simulink model "VCMGCM1962020b_v2"  (R2020b)
settings: Solver=FixedStepDiscrete  StartTime=0.0  StopTime=10.0  FixedStep=0.005  RelTol=1e-3  EnableMultiTasking=on
PreLoadFcn:
  | try, model_open; catch, disp('Error occurred while executing model pre-load callback: model_open.m'); disp('Please assure that the MATLAB working directory is set to the model directory before opening.'); end
InitFcn:
  | try, model_open; catch, end
undefined symbols (not defined in the file): Bridge, GCM, H, raptor_get_param_eval, raptor_get_safe_string, raptor_xcp_function
libraries: Blocks_lib x1165, Raptor_lib x665, simulink x62, VCM_lib x5
(part 19 of 23)

== system VCMGCM1962020b_v2/Fgnd/Sensors/CAN/Other/EPAS/EPASG7GenericFdbk2 ==
  DiagEnbl : Inport
  Bus Creator : BusCreator  Inputs=4
  CANRxField : Blocks_lib/CANRxField  typ='double'  custom=off  custom_nam=[nam '---']  custom_units='---'
  CANRxField1 : Blocks_lib/CANRxField  typ='double'  custom=off  custom_nam=[nam '---']  custom_units='---'
  CANRxField2 : Blocks_lib/CANRxField  typ='double'  custom=off  custom_nam=[nam '---']  custom_units='---'
  CANRxMsgStatus : Blocks_lib/CANRxMsgStatus  samptime=samptime  custom=on  custom_nam=[nam '---']  msgnam=EPASG7GenericFdbk2
  Header : Blocks_lib/Header  width=Landscape  addtext=''
  raptor_can_rxmsg : Raptor_lib/CAN/raptor_can_rxmsg  canDefinition=struct('dbcFile', 'EPAS_G7GenericExternal.dbc','message', 'G7GenericFdbk2','comment', '','signals', {{'FDBK2_Velocity','FDBK2_MotorTemperature','FDBK2_BoardTemperature'}},'enabled', [ 1 1 1;],'scaled', [ 1 1 1;],'canBus', 'bus','messageID', [ 419365651;],'idMask', [ 536870911;],'payloadMask', [],'payloadValue', [],'period', [ 0;],'mailbox', '[]','queueSize', [ 1;],'label', [ 1;],'ver', [ 2;],'showID', [ 0;],'showRaw', [ 0;],'fill', [ 0;],'editID', [ 0;],'signalOrder', [ 3;],'signalAscDes', [ 1;])  canBus=bus  mailbox=[]  payloadMask=[]  payloadValue=[]  idMask=hex2dec('1FFFFFFF')  queueSize=1  showID=0  label=1  fill=0  id=419365651  showRaw=0  showAge=1  signalOrder=3  signalInfo={{struct('Name', 'FDBK2_Velocity','Startbit', [ 0;],'SignalSize', [ 32;],'ByteOrder', 'LittleEndian','ValueType', 'SIGNED','Class', 'int32','Signed', [ 1;],'Factor', [ 9.5367e-07;],'Offset', [ 0;],'Min', [ -2048;],'Max', [ 2048;],'Units', 'RPM','Comment', '','StartBit', [ 0;]),struct('Name', 'FDBK2_MotorTemperature','Startbit', [ 0;],'SignalSize', [ 8;],'ByteOrder', 'LittleEndian','ValueType', 'UNSIGNED','Class', 'uint8','Signed', [ 0;],'Factor', [ 1;],'Offset', [ -40;],'Min', [ -40;],'Max', [ 215;],'Units', 'C','Comment', '','StartBit', [ 48;]),struct('Name', 'FDBK2_BoardTemperature','Startbit', [ 0;],'SignalSize', [ 8;],'ByteOrder', 'LittleEndian','ValueType', 'UNSIGNED','Class', 'uint8','Signed', [ 0;],'Factor', [ 1;],'Offset', [ -40;],'Min', [ -40;],'Max', [ 215;],'Units', 'C','Comment', '','StartBit', [ 32;])}}
      settings: SourceProductName=Raptor
  Data : Outport  VectorParamsAs1DForOutWhenUnconnected=off
  wires:
  Bus Creator/1 -> Data/1  "EPASG7GenericFdbk2"
  raptor_can_rxmsg/2 -> CANRxField/1  "FDBK2_Velocity"
  CANRxMsgStatus/1 -> Bus Creator/1
  CANRxField/1 -> Bus Creator/2
  DiagEnbl/1 -> CANRxMsgStatus/1
  raptor_can_rxmsg/1 -> CANRxMsgStatus/2  "Age"
  raptor_can_rxmsg/3 -> CANRxField1/1  "FDBK2_MotorTemperature"
  CANRxField1/1 -> Bus Creator/3
  raptor_can_rxmsg/4 -> CANRxField2/1  "FDBK2_BoardTemperature"
  CANRxField2/1 -> Bus Creator/4

== system VCMGCM1962020b_v2/Fgnd/Sensors/CAN/Other/EPAS/EPASG7GenericFdbk3 ==
  DiagEnbl : Inport
  Bus Creator : BusCreator  Inputs=3
  CANRxField : Blocks_lib/CANRxField  typ='double'  custom=off  custom_nam=[nam '---']  custom_units='---'
  CANRxField1 : Blocks_lib/CANRxField  typ='double'  custom=off  custom_nam=[nam '---']  custom_units='---'
  CANRxMsgStatus : Blocks_lib/CANRxMsgStatus  samptime=samptime  custom=on  custom_nam=[nam '---']  msgnam=EPASG7GenericFdbk3
  Header : Blocks_lib/Header  width=Landscape  addtext=''
  raptor_can_rxmsg : Raptor_lib/CAN/raptor_can_rxmsg  canDefinition=struct('dbcFile', 'EPAS_G7GenericExternal.dbc','message', 'G7GenericFdbk3','comment', '','signals', {{'FDBK3_TorqueIn','FDBK3_AssistCommand'}},'enabled', [ 1 1;],'scaled', [ 1 1;],'canBus', 'bus','messageID', [ 419365907;],'idMask', [ 536870911;],'payloadMask', [],'payloadValue', [],'period', [ 0;],'mailbox', '[]','queueSize', [ 1;],'label', [ 1;],'ver', [ 2;],'showID', [ 0;],'showRaw', [ 0;],'fill', [ 0;],'editID', [ 0;],'signalOrder', [ 3;],'signalAscDes', [ 1;])  canBus=bus  mailbox=[]  payloadMask=[]  payloadValue=[]  idMask=hex2dec('1FFFFFFF')  queueSize=1  showID=0  label=1  fill=0  id=419365907  showRaw=0  showAge=1  signalOrder=3  signalInfo={{struct('Name', 'FDBK3_TorqueIn','Startbit', [ 0;],'SignalSize', [ 32;],'ByteOrder', 'LittleEndian','ValueType', 'SIGNED','Class', 'int32','Signed', [ 1;],'Factor', [ 9.5367e-07;],'Offset', [ 0;],'Min', [ -2048;],'Max', [ 2048;],'Units', 'Nm','Comment', '','StartBit', [ 0;]),struct('Name', 'FDBK3_AssistCommand','Startbit', [ 0;],'SignalSize', [ 32;],'ByteOrder', 'LittleEndian','ValueType', 'SIGNED','Class', 'int32','Signed', [ 1;],'Factor', [ 9.5367e-07;],'Offset', [ 0;],'Min', [ -2048;],'Max', [ 2048;],'Units', '%','Comment', '','StartBit', [ 32;])}}
      settings: SourceProductName=Raptor
  Data : Outport  VectorParamsAs1DForOutWhenUnconnected=off
  wires:
  CANRxField1/1 -> Bus Creator/3
  raptor_can_rxmsg/3 -> CANRxField1/1  "FDBK3_AssistCommand"
  raptor_can_rxmsg/1 -> CANRxMsgStatus/2  "Age"
  DiagEnbl/1 -> CANRxMsgStatus/1
  CANRxField/1 -> Bus Creator/2
  CANRxMsgStatus/1 -> Bus Creator/1
  raptor_can_rxmsg/2 -> CANRxField/1  "FDBK3_TorqueIn"
  Bus Creator/1 -> Data/1  "EPASG7GenericFdbk3"

== system VCMGCM1962020b_v2/Fgnd/Sensors/CAN/Other/EPAS/EPASG7GenericFdbk4 ==
  DiagEnbl : Inport
  Bus Creator : BusCreator  Inputs=2
  CANRxField : Blocks_lib/CANRxField  typ='double'  custom=off  custom_nam=[nam '---']  custom_units='---'
  CANRxMsgStatus : Blocks_lib/CANRxMsgStatus  samptime=samptime  custom=on  custom_nam=[nam '---']  msgnam=EPASG7GenericFdbk4
  Header : Blocks_lib/Header  width=Landscape  addtext=''
  raptor_can_rxmsg : Raptor_lib/CAN/raptor_can_rxmsg  canDefinition=struct('dbcFile', 'EPAS_G7GenericExternal.dbc','message', 'G7GenericFdbk4','comment', '','signals', {{'FDBK4_P3','FDBK4_P2','FDBK4_P1','FDBK4_MessageCounter','FDBK4_CommandMode'}},'enabled', [ 0 0 0 0 1;],'scaled', [ 1 1 1 1 1;],'canBus', 'bus','messageID', [ 419366163;],'idMask', [ 536870911;],'payloadMask', [],'payloadValue', [],'period', [ 0;],'mailbox', '[]','queueSize', [ 1;],'label', [ 1;],'ver', [ 2;],'showID', [ 0;],'showRaw', [ 0;],'fill', [ 0;],'editID', [ 0;],'signalOrder', [ 3;],'signalAscDes', [ 1;])  canBus=bus  mailbox=[]  payloadMask=[]  payloadValue=[]  idMask=hex2dec('1FFFFFFF')  queueSize=1  showID=0  label=1  fill=0  id=419366163  showRaw=0  showAge=1  signalOrder=3  signalInfo={{struct('Name', 'FDBK4_P3','Startbit', [ 0;],'SignalSize', [ 16;],'ByteOrder', 'LittleEndian','ValueType', 'UNSIGNED','Class', 'uint16','Signed', [ 0;],'Factor', [ 1;],'Offset', [ 0;],'Min', [ 0;],'Max', [ 4095;],'Units', 'Counts','Comment', '','StartBit', [ 32;]),struct('Name', 'FDBK4_P2','Startbit', [ 0;],'SignalSize', [ 16;],'ByteOrder', 'LittleEndian','ValueType', 'UNSIGNED','Class', 'uint16','Signed', [ 0;],'Factor', [ 1;],'Offset', [ 0;],'Min', [ 0;],'Max', [ 4095;],'Units', 'Counts','Comment', '','StartBit', [ 16;]),struct('Name', 'FDBK4_P1','Startbit', [ 0;],'SignalSize', [ 16;],'ByteOrder', 'LittleEndian','ValueType', 'UNSIGNED','Class', 'uint16','Signed', [ 0;],'Factor', [ 1;],'Offset', [ 0;],'Min', [ 0;],'Max', [ 4095;],'Units', 'Counts','Comment', '','StartBit', [ 0;]),struct('Name', 'FDBK4_MessageCounter','Startbit', [ 0;],'SignalSize', [ 8;],'ByteOrder', 'LittleEndian','ValueType', 'UNSIGNED','Class', 'uint8','Signed', [ 0;],'Factor', [ 1;],'Offset', [ 0;],'Min', [ 0;],'Max', [ 255;],'Units', 'Count','Comment', '','StartBit', [ 56;]),struct('Name', 'FDBK4_CommandMode','Startbit', [ 0;],'SignalSize', [ 8;],'ByteOrder', 'LittleEndian','ValueType', 'UNSIGNED','Class', 'uint8','Signed', [ 0;],'Factor', [ 1;],'Offset', [ 0;],'Min', [ 0;],'Max', [ 0;],'Units', '','Comment', '','StartBit', [ 48;])}}
      settings: SourceProductName=Raptor
  Data : Outport  VectorParamsAs1DForOutWhenUnconnected=off
  wires:
  Bus Creator/1 -> Data/1  "EPASG7GenericFdbk4"
  raptor_can_rxmsg/2 -> CANRxField/1  "FDBK4_CommandMode"
  CANRxMsgStatus/1 -> Bus Creator/1
  CANRxField/1 -> Bus Creator/2
  DiagEnbl/1 -> CANRxMsgStatus/1
  raptor_can_rxmsg/1 -> CANRxMsgStatus/2  "Age"

== system VCMGCM1962020b_v2/Fgnd/Sensors/CAN/Other/EPAS/EPASG7GenericFdbk6 ==
  DiagEnbl : Inport
  Bus Creator : BusCreator  Inputs=3
  CANRxField : Blocks_lib/CANRxField  typ='double'  custom=off  custom_nam=[nam '---']  custom_units='---'
  CANRxField1 : Blocks_lib/CANRxField  typ='double'  custom=off  custom_nam=[nam '---']  custom_units='---'
  CANRxMsgStatus : Blocks_lib/CANRxMsgStatus  samptime=samptime  custom=on  custom_nam=[nam '---']  msgnam=EPASG7GenericFdbk6
  Header : Blocks_lib/Header  width=Landscape  addtext=''
  raptor_can_rxmsg : Raptor_lib/CAN/raptor_can_rxmsg  canDefinition=struct('dbcFile', 'EPAS_G7GenericExternal.dbc','message', 'G7GenericFdbk6','comment', '','signals', {{'FDBK6_Velocity','FDBK6_Position'}},'enabled', [ 1 1;],'scaled', [ 1 1;],'canBus', 'bus','messageID', [ 419373587;],'idMask', [ 536870911;],'payloadMask', [],'payloadValue', [],'period', [ 0;],'mailbox', '[]','queueSize', [ 1;],'label', [ 1;],'ver', [ 2;],'showID', [ 0;],'showRaw', [ 0;],'fill', [ 0;],'editID', [ 0;],'signalOrder', [ 3;],'signalAscDes', [ 1;])  canBus=bus  mailbox=[]  payloadMask=[]  payloadValue=[]  idMask=hex2dec('1FFFFFFF')  queueSize=1  showID=0  label=1  fill=0  id=419373587  showRaw=0  showAge=1  signalOrder=3  signalInfo={{struct('Name', 'FDBK6_Velocity','Startbit', [ 0;],'SignalSize', [ 32;],'ByteOrder', 'LittleEndian','ValueType', 'SIGNED','Class', 'int32','Signed', [ 1;],'Factor', [ 3.8147e-06;],'Offset', [ 0;],'Min', [ -8192;],'Max', [ 8192;],'Units', 'RPM','Comment', '','StartBit', [ 32;]),struct('Name', 'FDBK6_Position','Startbit', [ 0;],'SignalSize', [ 32;],'ByteOrder', 'LittleEndian','ValueType', 'SIGNED','Class', 'int32','Signed', [ 1;],'Factor', [ 3.8147e-06;],'Offset', [ 0;],'Min', [ -8192;],'Max', [ 8192;],'Units', 'DEG','Comment', '','StartBit', [ 0;])}}
      settings: SourceProductName=Raptor
  Data : Outport  VectorParamsAs1DForOutWhenUnconnected=off
  wires:
  raptor_can_rxmsg/1 -> CANRxMsgStatus/2  "Age"
  DiagEnbl/1 -> CANRxMsgStatus/1
  CANRxField/1 -> Bus Creator/2
  CANRxMsgStatus/1 -> Bus Creator/1
  raptor_can_rxmsg/2 -> CANRxField/1  "FDBK6_Velocity"
  Bus Creator/1 -> Data/1  "EPASG7GenericFdbk6"
  raptor_can_rxmsg/3 -> CANRxField1/1  "FDBK6_Position"
  CANRxField1/1 -> Bus Creator/3

== system VCMGCM1962020b_v2/Fgnd/Sensors/CAN/Other/EPAS/EPASG7GenericFdbk7 ==
  DiagEnbl : Inport
  Bus Creator : BusCreator  Inputs=3
  CANRxField : Blocks_lib/CANRxField  typ='double'  custom=off  custom_nam=[nam '---']  custom_units='---'
  CANRxField1 : Blocks_lib/CANRxField  typ='double'  custom=off  custom_nam=[nam '---']  custom_units='---'
  CANRxMsgStatus : Blocks_lib/CANRxMsgStatus  samptime=samptime  custom=on  custom_nam=[nam '---']  msgnam=EPASG7GenericFdbk7
  Header : Blocks_lib/Header  width=Landscape  addtext=''
  raptor_can_rxmsg : Raptor_lib/CAN/raptor_can_rxmsg  canDefinition=struct('dbcFile', 'EPAS_G7GenericExternal.dbc','message', 'G7GenericFdbk7','comment', '','signals', {{'FDBK7_QAxisCurrent','FDBK7_DAxisCurrent'}},'enabled', [ 1 1;],'scaled', [ 1 1;],'canBus', 'bus','messageID', [ 419373843;],'idMask', [ 536870911;],'payloadMask', [],'payloadValue', [],'period', [ 0;],'mailbox', '[]','queueSize', [ 1;],'label', [ 1;],'ver', [ 2;],'showID', [ 0;],'showRaw', [ 0;],'fill', [ 0;],'editID', [ 0;],'signalOrder', [ 3;],'signalAscDes', [ 1;])  canBus=bus  mailbox=[]  payloadMask=[]  payloadValue=[]  idMask=hex2dec('1FFFFFFF')  queueSize=1  showID=0  label=1  fill=0  id=419373843  showRaw=0  showAge=1  signalOrder=3  signalInfo={{struct('Name', 'FDBK7_QAxisCurrent','Startbit', [ 0;],'SignalSize', [ 32;],'ByteOrder', 'LittleEndian','ValueType', 'SIGNED','Class', 'int32','Signed', [ 1;],'Factor', [ 3.8147e-06;],'Offset', [ 0;],'Min', [ -8192;],'Max', [ 8192;],'Units', 'A','Comment', '','StartBit', [ 0;]),struct('Name', 'FDBK7_DAxisCurrent','Startbit', [ 0;],'SignalSize', [ 32;],'ByteOrder', 'LittleEndian','ValueType', 'SIGNED','Class', 'int32','Signed', [ 1;],'Factor', [ 3.8147e-06;],'Offset', [ 0;],'Min', [ -8192;],'Max', [ 8192;],'Units', 'A','Comment', '','StartBit', [ 32;])}}
      settings: SourceProductName=Raptor
  Data : Outport  VectorParamsAs1DForOutWhenUnconnected=off
  wires:
  CANRxField1/1 -> Bus Creator/3
  raptor_can_rxmsg/3 -> CANRxField1/1  "FDBK7_DAxisCurrent"
  Bus Creator/1 -> Data/1  "EPASG7GenericFdbk7"
  raptor_can_rxmsg/2 -> CANRxField/1  "FDBK7_QAxisCurrent"
  CANRxMsgStatus/1 -> Bus Creator/1
  CANRxField/1 -> Bus Creator/2
  DiagEnbl/1 -> CANRxMsgStatus/1
  raptor_can_rxmsg/1 -> CANRxMsgStatus/2  "Age"

== system VCMGCM1962020b_v2/Fgnd/Sensors/CAN/Other/EPAS/EPASG7GenericFdbk8 ==
  DiagEnbl : Inport
  Bus Creator : BusCreator  Inputs=2
  CANRxField : Blocks_lib/CANRxField  typ='double'  custom=off  custom_nam=[nam '---']  custom_units='---'
  CANRxMsgStatus : Blocks_lib/CANRxMsgStatus  samptime=samptime  custom=on  custom_nam=[nam '---']  msgnam=EPASG7GenericFdbk8
  Header : Blocks_lib/Header  width=Landscape  addtext=''
  raptor_can_rxmsg : Raptor_lib/CAN/raptor_can_rxmsg  canDefinition=struct('dbcFile', 'EPAS_G7GenericExternal.dbc','message', 'G7GenericFdbk8','comment', '','signals', {{'FDBK8_RawPosition'}},'enabled', [ 1;],'scaled', [ 1;],'canBus', 'bus','messageID', [ 419374099;],'idMask', [ 536870911;],'payloadMask', [],'payloadValue', [],'period', [ 0;],'mailbox', '[]','queueSize', [ 1;],'label', [ 1;],'ver', [ 2;],'showID', [ 0;],'showRaw', [ 0;],'fill', [ 0;],'editID', [ 0;],'signalOrder', [ 3;],'signalAscDes', [ 1;])  canBus=bus  mailbox=[]  payloadMask=[]  payloadValue=[]  idMask=hex2dec('1FFFFFFF')  queueSize=1  showID=0  label=1  fill=0  id=419374099  showRaw=0  showAge=1  signalOrder=3  signalInfo={{struct('Name', 'FDBK8_RawPosition','Startbit', [ 0;],'SignalSize', [ 32;],'ByteOrder', 'LittleEndian','ValueType', 'SIGNED','Class', 'int32','Signed', [ 1;],'Factor', [ 3.8147e-06;],'Offset', [ 0;],'Min', [ -8192;],'Max', [ 8192;],'Units', 'DEG','Comment', '','StartBit', [ 0;])}}
      settings: SourceProductName=Raptor
  Data : Outport  VectorParamsAs1DForOutWhenUnconnected=off
  wires:
  raptor_can_rxmsg/1 -> CANRxMsgStatus/2  "Age"
  DiagEnbl/1 -> CANRxMsgStatus/1
  CANRxField/1 -> Bus Creator/2
  CANRxMsgStatus/1 -> Bus Creator/1
  raptor_can_rxmsg/2 -> CANRxField/1  "FDBK8_RawPosition"
  Bus Creator/1 -> Data/1  "EPASG7GenericFdbk8"

== system VCMGCM1962020b_v2/Fgnd/Sensors/CAN/Other/EPAS/EPASG7GenericFdbk9 ==
  DiagEnbl : Inport
  Bus Creator : BusCreator  Inputs=2
  CANRxField : Blocks_lib/CANRxField  typ='double'  custom=off  custom_nam=[nam '---']  custom_units='---'
  CANRxMsgStatus : Blocks_lib/CANRxMsgStatus  samptime=samptime  custom=on  custom_nam=[nam '---']  msgnam=EPASG7GenericFdbk9
  Header : Blocks_lib/Header  width=Landscape  addtext=''
  raptor_can_rxmsg : Raptor_lib/CAN/raptor_can_rxmsg  canDefinition=struct('dbcFile', 'EPAS_G7GenericExternal.dbc','message', 'G7GenericFdbk9','comment', '','signals', {{'FDBK9_MessageCounter','FDBK9_CommandVariable2','FDBK9_CommandVariable1','FDBK9_CommandMode'}},'enabled', [ 0 0 0 1;],'scaled', [ 1 1 1 1;],'canBus', 'bus','messageID', [ 419374355;],'idMask', [ 536870911;],'payloadMask', [],'payloadValue', [],'period', [ 0;],'mailbox', '[]','queueSize', [ 1;],'label', [ 1;],'ver', [ 2;],'showID', [ 0;],'showRaw', [ 0;],'fill', [ 0;],'editID', [ 0;],'signalOrder', [ 3;],'signalAscDes', [ 1;])  canBus=bus  mailbox=[]  payloadMask=[]  payloadValue=[]  idMask=hex2dec('1FFFFFFF')  queueSize=1  showID=0  label=1  fill=0  id=419374355  showRaw=0  showAge=1  signalOrder=3  signalInfo={{struct('Name', 'FDBK9_MessageCounter','Startbit', [ 0;],'SignalSize', [ 8;],'ByteOrder', 'LittleEndian','ValueType', 'UNSIGNED','Class', 'uint8','Signed', [ 0;],'Factor', [ 1;],'Offset', [ 0;],'Min', [ 0;],'Max', [ 255;],'Units', 'Count','Comment', '','StartBit', [ 8;]),struct('Name', 'FDBK9_CommandVariable2','Startbit', [ 0;],'SignalSize', [ 16;],'ByteOrder', 'LittleEndian','ValueType', 'SIGNED','Class', 'int16','Signed', [ 1;],'Factor', [ 0.0039063;],'Offset', [ 0;],'Min', [ -128;],'Max', [ 127.9961;],'Units', '','Comment', '','StartBit', [ 48;]),struct('Name', 'FDBK9_CommandVariable1','Startbit', [ 0;],'SignalSize', [ 32;],'ByteOrder', 'LittleEndian','ValueType', 'SIGNED','Class', 'int32','Signed', [ 1;],'Factor', [ 3.8147e-06;],'Offset', [ 0;],'Min', [ -8192;],'Max', [ 8192;],'Units', '','Comment', '','StartBit', [ 16;]),struct('Name', 'FDBK9_CommandMode','Startbit', [ 0;],'SignalSize', [ 8;],'ByteOrder', 'LittleEndian','ValueType', 'UNSIGNED','Class', 'uint8','Signed', [ 0;],'Factor', [ 1;],'Offset', [ 0;],'Min', [ 0;],'Max', [ 0;],'Units', '','Comment', '','StartBit', [ 0;])}}
      settings: SourceProductName=Raptor
  Data : Outport  VectorParamsAs1DForOutWhenUnconnected=off
  wires:
  Bus Creator/1 -> Data/1  "EPASG7GenericFdbk9"
  CANRxMsgStatus/1 -> Bus Creator/1
  CANRxField/1 -> Bus Creator/2
  DiagEnbl/1 -> CANRxMsgStatus/1
  raptor_can_rxmsg/1 -> CANRxMsgStatus/2  "Age"
  raptor_can_rxmsg/2 -> CANRxField/1  "FDBK9_CommandMode"

== system VCMGCM1962020b_v2/Fgnd/Sensors/CAN/Other/Heater/HTR_OUT_2 ==
  DiagEnbl : Inport
  Bus Creator : BusCreator  Inputs=7
  CANRxField{,1..5} (6 alike) : Blocks_lib/CANRxField  typ='double'  custom=off  custom_nam='---'  custom_units='---'
  CANRxMsgStatus : Blocks_lib/CANRxMsgStatus  samptime=samptime  custom=off  custom_nam='Name'  msgnam=HTR_OUT_2
  Header : Blocks_lib/Header  width=Landscape  addtext=''
  raptor_can_rxmsg : Raptor_lib/CAN/raptor_can_rxmsg  canDefinition=struct('dbcFile', 'ATSS17002_EWH40Dx-245.dbc','message', 'HTR_OUT_2','comment', '','signals', {{'IGBT_Q11_SNSR','IGBT_Q12_SNSR','IGBT_Q13_SNSR','IGBT_Q14_SNSR','BOARD_SNSR','HV_VOLT_DC'}},'enabled', [ 1 1 1 1 1 1;],'canBus', 'bus','messageID', [ 693;],'idMask', [ 536870911;],'payloadMask', [],'payloadValue', [],'period', [ 0;],'mailbox', '''''','queueSize', [ 1;],'label', [ 1;],'ver', [ 2;],'showID', [ 0;],'showRaw', [ 0;],'fill', [ 0;],'editID', [ 0;],'signalOrder', [ 3;])  canBus=bus  mailbox=''  payloadMask=[]  payloadValue=[]  idMask=hex2dec('1FFFFFFF')  queueSize=1  showID=0  label=1  fill=0  id=693  showRaw=0  showAge=1  signalOrder=3  signalInfo={{struct('Name', 'IGBT_Q11_SNSR','Startbit', [ 0;],'SignalSize', [ 8;],'ByteOrder', 'BigEndian','ValueType', 'UNSIGNED','Class', 'uint8','Signed', [ 0;],'Factor', [ 1;],'Offset', [ -40;],'Min', [ -40;],'Max', [ 150;],'Units', 'degC','Comment', 'IGBT Q11 Temperature Sensor','StartBit', [ 0;]),struct('Name', 'IGBT_Q12_SNSR','Startbit', [ 0;],'SignalSize', [ 8;],'ByteOrder', 'BigEndian','ValueType', 'UNSIGNED','Class', 'uint8','Signed', [ 0;],'Factor', [ 1;],'Offset', [ -40;],'Min', [ -40;],'Max', [ 150;],'Units', 'degC','Comment', 'IGBT Q12 Temperature Sensor','StartBit', [ 8;]),struct('Name', 'IGBT_Q13_SNSR','Startbit', [ 0;],'SignalSize', [ 8;],'ByteOrder', 'BigEndian','ValueType', 'UNSIGNED','Class', 'uint8','Signed', [ 0;],'Factor', [ 1;],'Offset', [ -40;],'Min', [ -40;],'Max', [ 150;],'Units', 'degC','Comment', 'IGBT Q13 Temperature Sensor','StartBit', [ 16;]),struct('Name', 'IGBT_Q14_SNSR','Startbit', [ 0;],'SignalSize', [ 8;],'ByteOrder', 'BigEndian','ValueType', 'UNSIGNED','Class', 'uint8','Signed', [ 0;],'Factor', [ 1;],'Offset', [ -40;],'Min', [ -40;],'Max', [ 150;],'Units', 'degC','Comment', 'IGBT Q14 Temperature Sensor','StartBit', [ 24;]),struct('Name', 'BOARD_SNSR','Startbit', [ 0;],'SignalSize', [ 8;],'ByteOrder', 'BigEndian','ValueType', 'UNSIGNED','Class', 'uint8','Signed', [ 0;],'Factor', [ 1;],'Offset', [ -40;],'Min', [ -40;],'Max', [ 150;],'Units', 'degC','Comment', 'Circuit Board Temperature Sensor','StartBit', [ 32;]),struct('Name', 'HV_VOLT_DC','Startbit', [ 0;],'SignalSize', [ 8;],'ByteOrder', 'BigEndian','ValueType', 'UNSIGNED','Class', 'uint8','Signed', [ 0;],'Factor', [ 2.5;],'Offset', [ 0;],'Min', [ 0;],'Max', [ 555;],'Units', 'V','Comment', 'Heater Electric Voltage','StartBit', [ 40;])}}
      settings: SourceProductName=Raptor
  Data : Outport  VectorParamsAs1DForOutWhenUnconnected=off
  wires:
  raptor_can_rxmsg/3 -> CANRxField1/1  "IGBT_Q12_SNSR"
  raptor_can_rxmsg/2 -> CANRxField/1  "IGBT_Q11_SNSR"
  Bus Creator/1 -> Data/1  "MsgName"
  raptor_can_rxmsg/4 -> CANRxField2/1  "IGBT_Q13_SNSR"
  raptor_can_rxmsg/5 -> CANRxField3/1  "IGBT_Q14_SNSR"
  raptor_can_rxmsg/6 -> CANRxField4/1  "BOARD_SNSR"
  raptor_can_rxmsg/7 -> CANRxField5/1  "HV_VOLT_DC"
  CANRxField5/1 -> Bus Creator/7
  CANRxField4/1 -> Bus Creator/6
  CANRxField3/1 -> Bus Creator/5
  CANRxField2/1 -> Bus Creator/4
  CANRxField1/1 -> Bus Creator/3
  CANRxField/1 -> Bus Creator/2
  CANRxMsgStatus/1 -> Bus Creator/1
  DiagEnbl/1 -> CANRxMsgStatus/1
  raptor_can_rxmsg/1 -> CANRxMsgStatus/2  "Age"

== system VCMGCM1962020b_v2/Fgnd/Sensors/CAN/Other/Heater/MsgName ==
  DiagEnbl : Inport
  Bus Creator : BusCreator  Inputs=8
  CANRxField : Blocks_lib/CANRxField  typ='boolean'  custom=off  custom_nam='---'  custom_units='---'
  CANRxField1 : Blocks_lib/CANRxField  typ='boolean'  custom=off  custom_nam='---'  custom_units='---'
  CANRxField{2..5} (4 alike) : Blocks_lib/CANRxField  typ='double'  custom=off  custom_nam='---'  custom_units='---'
  CANRxField6 : Blocks_lib/CANRxField  typ='uint16'  custom=off  custom_nam='---'  custom_units='---'
  CANRxMsgStatus : Blocks_lib/CANRxMsgStatus  samptime=samptime  custom=off  custom_nam='Name'  msgnam=HTR_OUT_1
  Header : Blocks_lib/Header  width=Landscape  addtext=''
  raptor_can_rxmsg : Raptor_lib/CAN/raptor_can_rxmsg  canDefinition=struct('dbcFile', 'ATSS17002_EWH40Dx-245.dbc','message', 'HTR_OUT_1','comment', '','signals', {{'HTR_PWR_REQ_FLAG','BUS_OFF_HTR','HTR_PWR_AC','HTR_CURRENT','HTR_W_IN_SNSR','HTR_W_OUT_SNSR','HTR_STAT'}},'enabled', [ 1 1 1 1 1 1 1;],'canBus', 'bus','messageID', [ 692;],'idMask', [ 536870911;],'payloadMask', [],'payloadValue', [],'period', [ 0;],'mailbox', '''''','queueSize', [ 1;],'label', [ 1;],'ver', [ 2;],'showID', [ 0;],'showRaw', [ 0;],'fill', [ 0;],'editID', [ 0;],'signalOrder', [ 3;],'signalAscDes', [ 1;])  canBus=bus  mailbox=''  payloadMask=[]  payloadValue=[]  idMask=hex2dec('1FFFFFFF')  queueSize=1  showID=0  label=1  fill=0  id=692  showRaw=0  showAge=1  signalOrder=3  signalInfo={{struct('Name', 'HTR_PWR_REQ_FLAG','Startbit', [ 0;],'SignalSize', [ 1;],'ByteOrder', 'BigEndian','ValueType', 'UNSIGNED','Class', 'uint8','Signed', [ 0;],'Factor', [ 1;],'Offset', [ 0;],'Min', [ 0;],'Max', [ 1;],'Units', '','Comment', 'LV Power Keep Request Flag','StartBit', [ 0;]),struct('Name', 'BUS_OFF_HTR','Startbit', [ 0;],'SignalSize', [ 1;],'ByteOrder', 'BigEndian','ValueType', 'UNSIGNED','Class', 'uint8','Signed', [ 0;],'Factor', [ 1;],'Offset', [ 0;],'Min', [ 0;],'Max', [ 1;],'Units', '','Comment', 'Bus off flag','StartBit', [ 1;]),struct('Name', 'HTR_PWR_AC','Startbit', [ 0;],'SignalSize', [ 8;],'ByteOrder', 'BigEndian','ValueType', 'UNSIGNED','Class', 'uint8','Signed', [ 0;],'Factor', [ 40;],'Offset', [ 0;],'Min', [ 0;],'Max', [ 10160;],'Units', 'W','Comment', 'Heater Power','StartBit', [ 8;]),struct('Name', 'HTR_CURRENT','Startbit', [ 0;],'SignalSize', [ 8;],'ByteOrder', 'BigEndian','ValueType', 'UNSIGNED','Class', 'uint8','Signed', [ 0;],'Factor', [ 0.2;],'Offset', [ 0;],'Min', [ 0;],'Max', [ 50;],'Units', 'A','Comment', 'Heater Electric Current','StartBit', [ 16;]),struct('Name', 'HTR_W_IN_SNSR','Startbit', [ 0;],'SignalSize', [ 8;],'ByteOrder', 'BigEndian','ValueType', 'UNSIGNED','Class', 'uint8','Signed', [ 0;],'Factor', [ 1;],'Offset', [ -40;],'Min', [ -40;],'Max', [ 214;],'Units', 'degC','Comment', 'Heater Water Inlet Sensor','StartBit', [ 24;]),struct('Name', 'HTR_W_OUT_SNSR','Startbit', [ 0;],'SignalSize', [ 8;],'ByteOrder', 'BigEndian','ValueType', 'UNSIGNED','Class', 'uint8','Signed', [ 0;],'Factor', [ 1;],'Offset', [ -40;],'Min', [ -40;],'Max', [ 214;],'Units', 'degC','Comment', 'Heater Water Outlet Sensor','StartBit', [ 32;]),struct('Name', 'HTR_STAT','Startbit', [ 0;],'SignalSize', [ 16;],'ByteOrder', 'BigEndian','ValueType', 'UNSIGNED','Class', 'uint16','Signed', [ 0;],'Factor', [ 1;],'Offset', [ 0;],'Min', [ 0;],'Max', [ 65535;],'Units', '','Comment', 'Heater Status (see Technical Information document for bit field definition)','StartBit', [ 48;])}}
      settings: SourceProductName=Raptor
  Data : Outport  VectorParamsAs1DForOutWhenUnconnected=off
  wires:
  raptor_can_rxmsg/8 -> CANRxField6/1  "HTR_STAT"
  raptor_can_rxmsg/7 -> CANRxField5/1  "HTR_W_OUT_SNSR"
  raptor_can_rxmsg/6 -> CANRxField4/1  "HTR_W_IN_SNSR"
  raptor_can_rxmsg/5 -> CANRxField3/1  "HTR_CURRENT"
  raptor_can_rxmsg/4 -> CANRxField2/1  "HTR_PWR_AC"
  raptor_can_rxmsg/3 -> CANRxField1/1  "BUS_OFF_HTR"
  raptor_can_rxmsg/2 -> CANRxField/1  "HTR_PWR_REQ_FLAG"
  Bus Creator/1 -> Data/1  "MsgName"
  CANRxField6/1 -> Bus Creator/8
  CANRxField5/1 -> Bus Creator/7
  CANRxField4/1 -> Bus Creator/6
  CANRxField3/1 -> Bus Creator/5
  CANRxField2/1 -> Bus Creator/4
  CANRxField1/1 -> Bus Creator/3
  CANRxField/1 -> Bus Creator/2
  CANRxMsgStatus/1 -> Bus Creator/1
  DiagEnbl/1 -> CANRxMsgStatus/1
  raptor_can_rxmsg/1 -> CANRxMsgStatus/2  "Age"

== system VCMGCM1962020b_v2/Fgnd/Sensors/CAN/Other/Power Steering Pump Inverter/MsgName ==
  DiagEnbl : Inport
  Bus Creator : BusCreator  Inputs=4
  CANRxField : Blocks_lib/CANRxField  typ='double'  custom=on  custom_nam=[nam '---']  custom_units='---'
  CANRxField1 : Blocks_lib/CANRxField  typ='double'  custom=on  custom_nam=[nam '---']  custom_units='---'
  CANRxField2 : Blocks_lib/CANRxField  typ='double'  custom=on  custom_nam=[nam '---']  custom_units='---'
  CANRxMsgStatus : Blocks_lib/CANRxMsgStatus  samptime=samptime  custom=on  custom_nam=[nam '---']  msgnam=PSPInvtrHS1_Torque_Feedback
  Header : Blocks_lib/Header  width=Landscape  addtext=''
  raptor_can_rxmsg : Raptor_lib/CAN/raptor_can_rxmsg  canDefinition=struct('dbcFile', 'SevconInverter_H_Protocol.dbc','message', 'HS1_Torque_Feedback','comment', '','signals', {{'DC_Link_Current','Speed_Measured','SEQ_Torque','CS_Torque','Torque_Measured'}},'enabled', [ 1 1 0 0 1;],'canBus', 'bus','messageID', [ 421068544;],'idMask', [ 536870656;],'payloadMask', [],'payloadValue', [],'period', [ 0;],'mailbox', 'msgnam','queueSize', [ 1;],'label', [ 1;],'ver', [ 2;],'showID', [ 0;],'showRaw', [ 0;],'fill', [ 0;],'editID', [ 0;],'signalOrder', [ 3;])  canBus=bus  mailbox=msgnam  payloadMask=[]  payloadValue=[]  idMask=hex2dec('1FFFFF00')  queueSize=1  showID=0  label=1  fill=0  id=421068544  showRaw=0  showAge=1  signalOrder=3  signalInfo={{struct('Name', 'DC_Link_Current','Startbit', [ 0;],'SignalSize', [ 16;],'ByteOrder', 'LittleEndian','ValueType', 'SIGNED','Class', 'int16','Signed', [ 1;],'Factor', [ 1;],'Offset', [ 0;],'Min', [ -32768;],'Max', [ 32767;],'Units', 'A','Comment', '','StartBit', [ 32;]),struct('Name', 'Speed_Measured','Startbit', [ 0;],'SignalSize', [ 16;],'ByteOrder', 'LittleEndian','ValueType', 'SIGNED','Class', 'int16','Signed', [ 1;],'Factor', [ 1;],'Offset', [ 0;],'Min', [ -32768;],'Max', [ 32767;],'Units', 'RPM','Comment', '','StartBit', [ 16;]),struct('Name', 'SEQ_Torque','Startbit', [ 0;],'SignalSize', [ 8;],'ByteOrder', 'LittleEndian','ValueType', 'UNSIGNED','Class', 'uint8','Signed', [ 0;],'Factor', [ 1;],'Offset', [ 0;],'Min', [ 0;],'Max', [ 255;],'Units', '','Comment', '','StartBit', [ 48;]),struct('Name', 'CS_Torque','Startbit', [ 0;],'SignalSize', [ 8;],'ByteOrder', 'LittleEndian','ValueType', 'UNSIGNED','Class', 'uint8','Signed', [ 0;],'Factor', [ 1;],'Offset', [ 0;],'Min', [ 0;],'Max', [ 255;],'Units', '','Comment', '','StartBit', [ 56;]),struct('Name', 'Torque_Measured','Startbit', [ 0;],'SignalSize', [ 16;],'ByteOrder', 'LittleEndian','ValueType', 'SIGNED','Class', 'int16','Signed', [ 1;],'Factor', [ 0.0625;],'Offset', [ 0;],'Min', [ 0;],'Max', [ 0;],'Units', 'Nm','Comment', '','StartBit', [ 0;])}}
      settings: SourceProductName=Raptor
  Data : Outport  VectorParamsAs1DForOutWhenUnconnected=off
  wires:
  raptor_can_rxmsg/4 -> CANRxField2/1  "Torque_Measured"
  raptor_can_rxmsg/3 -> CANRxField1/1  "Speed_Measured"
  raptor_can_rxmsg/2 -> CANRxField/1  "DC_Link_Current"
  Bus Creator/1 -> Data/1  "MsgName"
  CANRxField2/1 -> Bus Creator/4
  CANRxField1/1 -> Bus Creator/3
  CANRxField/1 -> Bus Creator/2
  CANRxMsgStatus/1 -> Bus Creator/1
  DiagEnbl/1 -> CANRxMsgStatus/1
  raptor_can_rxmsg/1 -> CANRxMsgStatus/2  "Age"

== system VCMGCM1962020b_v2/Fgnd/Sensors/CAN/Other/Power Steering Pump Inverter/PSPInvtrHS2_Status_Feedback ==
  DiagEnbl : Inport
  Bus Creator : BusCreator  Inputs=5
  CANRxField : Blocks_lib/CANRxField  typ='uint8'  custom=on  custom_nam=[nam '---']  custom_units='---'
  CANRxField1 : Blocks_lib/CANRxField  typ='double'  custom=on  custom_nam=[nam '---']  custom_units='---'
  CANRxField2 : Blocks_lib/CANRxField  typ='double'  custom=on  custom_nam=[nam '---']  custom_units='---'
  CANRxField3 : Blocks_lib/CANRxField  typ='uint8'  custom=on  custom_nam=[nam '---']  custom_units='---'
  CANRxMsgStatus : Blocks_lib/CANRxMsgStatus  samptime=samptime  custom=on  custom_nam=[nam '---']  msgnam=PSPInvtrHS2_Status_Feedback
  Header : Blocks_lib/Header  width=Landscape  addtext=''
  raptor_can_rxmsg : Raptor_lib/CAN/raptor_can_rxmsg  canDefinition=struct('dbcFile', 'SevconInverter_H_Protocol.dbc','message', 'HS2_Status_Feedback','comment', '','signals', {{'Torque_Limit_Code','Torque_Available_Reverse','Torque_Available_Forward','SEQ_Status','CS_Status','InverterStatus'}},'enabled', [ 1 1 1 0 0 1;],'canBus', 'bus','messageID', [ 421134080;],'idMask', [ 536870656;],'payloadMask', [],'payloadValue', [],'period', [ 0;],'mailbox', 'msgnam','queueSize', [ 1;],'label', [ 1;],'ver', [ 2;],'showID', [ 0;],'showRaw', [ 0;],'fill', [ 0;],'editID', [ 0;],'signalOrder', [ 3;])  canBus=bus  mailbox=msgnam  payloadMask=[]  payloadValue=[]  idMask=hex2dec('1FFFFF00')  queueSize=1  showID=0  label=1  fill=0  id=421134080  showRaw=0  showAge=1  signalOrder=3  signalInfo={{struct('Name', 'Torque_Limit_Code','Startbit', [ 0;],'SignalSize', [ 8;],'ByteOrder', 'LittleEndian','ValueType', 'UNSIGNED','Class', 'uint8','Signed', [ 0;],'Factor', [ 1;],'Offset', [ 0;],'Min', [ 0;],'Max', [ 255;],'Units', '','Comment', '','StartBit', [ 40;]),struct('Name', 'Torque_Available_Reverse','Startbit', [ 0;],'SignalSize', [ 16;],'ByteOrder', 'LittleEndian','ValueType', 'SIGNED','Class', 'int16','Signed', [ 1;],'Factor', [ 0.0625;],'Offset', [ 0;],'Min', [ 0;],'Max', [ 0;],'Units', 'Nm','Comment', '','StartBit', [ 16;]),struct('Name', 'Torque_Available_Forward','Startbit', [ 0;],'SignalSize', [ 16;],'ByteOrder', 'LittleEndian','ValueType', 'SIGNED','Class', 'int16','Signed', [ 1;],'Factor', [ 0.0625;],'Offset', [ 0;],'Min', [ 0;],'Max', [ 0;],'Units', 'Nm','Comment', '','StartBit', [ 0;]),struct('Name', 'SEQ_Status','Startbit', [ 0;],'SignalSize', [ 8;],'ByteOrder', 'LittleEndian','ValueType', 'UNSIGNED','Class', 'uint8','Signed', [ 0;],'Factor', [ 1;],'Offset', [ 0;],'Min', [ 0;],'Max', [ 255;],'Units', '','Comment', '','StartBit', [ 48;]),struct('Name', 'CS_Status','Startbit', [ 0;],'SignalSize', [ 8;],'ByteOrder', 'LittleEndian','ValueType', 'UNSIGNED','Class', 'uint8','Signed', [ 0;],'Factor', [ 1;],'Offset', [ 0;],'Min', [ 0;],'Max', [ 255;],'Units', '','Comment', '','StartBit', [ 56;]),struct('Name', 'InverterStatus','Startbit', [ 0;],'SignalSize', [ 8;],'ByteOrder', 'LittleEndian','ValueType', 'UNSIGNED','Class', 'uint8','Signed', [ 0;],'Factor', [ 1;],'Offset', [ 0;],'Min', [ 0;],'Max', [ 255;],'Units', 'enum','Comment', '','StartBit', [ 32;])}}
      settings: SourceProductName=Raptor
  Data : Outport  VectorParamsAs1DForOutWhenUnconnected=off
  wires:
  raptor_can_rxmsg/5 -> CANRxField3/1  "InverterStatus"
  Bus Creator/1 -> Data/1  "MsgName"
  raptor_can_rxmsg/2 -> CANRxField/1  "Torque_Limit_Code"
  raptor_can_rxmsg/3 -> CANRxField1/1  "Torque_Available_Reverse"
  raptor_can_rxmsg/4 -> CANRxField2/1  "Torque_Available_Forward"
  CANRxField3/1 -> Bus Creator/5
  CANRxField2/1 -> Bus Creator/4
  CANRxField1/1 -> Bus Creator/3
  CANRxField/1 -> Bus Creator/2
  CANRxMsgStatus/1 -> Bus Creator/1
  DiagEnbl/1 -> CANRxMsgStatus/1
  raptor_can_rxmsg/1 -> CANRxMsgStatus/2  "Age"

== system VCMGCM1962020b_v2/Fgnd/Sensors/CAN/Other/Power Steering Pump Inverter/PSPInvtrHS3_Temperature_Feedback ==
  DiagEnbl : Inport
  Bus Creator : BusCreator  Inputs=4
  CANRxField : Blocks_lib/CANRxField  typ='double'  custom=on  custom_nam=[nam '---']  custom_units='---'
  CANRxField1 : Blocks_lib/CANRxField  typ='double'  custom=on  custom_nam=[nam '---']  custom_units='---'
  CANRxField2 : Blocks_lib/CANRxField  typ='double'  custom=on  custom_nam=[nam '---']  custom_units='---'
  CANRxMsgStatus : Blocks_lib/CANRxMsgStatus  samptime=samptime  custom=on  custom_nam=[nam '---']  msgnam=PSPInvtrHS3_Temperature_Feedback
  Header : Blocks_lib/Header  width=Landscape  addtext=''
  raptor_can_rxmsg : Raptor_lib/CAN/raptor_can_rxmsg  canDefinition=struct('dbcFile', 'SevconInverter_H_Protocol.dbc','message', 'HS3_Temperature_Feedback','comment', '','signals', {{'DC_Link_Voltage','SEQ_Temp','CS_Temp','MotorTempRemaining','InverterTempRemaining'}},'enabled', [ 1 0 0 1 1;],'canBus', 'bus','messageID', [ 421199616;],'idMask', [ 536870656;],'payloadMask', [],'payloadValue', [],'period', [ 0;],'mailbox', 'msgnam','queueSize', [ 1;],'label', [ 1;],'ver', [ 2;],'showID', [ 0;],'showRaw', [ 0;],'fill', [ 0;],'editID', [ 0;],'signalOrder', [ 3;])  canBus=bus  mailbox=msgnam  payloadMask=[]  payloadValue=[]  idMask=hex2dec('1FFFFF00')  queueSize=1  showID=0  label=1  fill=0  id=421199616  showRaw=0  showAge=1  signalOrder=3  signalInfo={{struct('Name', 'DC_Link_Voltage','Startbit', [ 0;],'SignalSize', [ 16;],'ByteOrder', 'LittleEndian','ValueType', 'SIGNED','Class', 'int16','Signed', [ 1;],'Factor', [ 0.0625;],'Offset', [ 0;],'Min', [ -2048;],'Max', [ 2047.9375;],'Units', 'V','Comment', '','StartBit', [ 32;]),struct('Name', 'SEQ_Temp','Startbit', [ 0;],'SignalSize', [ 8;],'ByteOrder', 'LittleEndian','ValueType', 'UNSIGNED','Class', 'uint8','Signed', [ 0;],'Factor', [ 1;],'Offset', [ 0;],'Min', [ 0;],'Max', [ 255;],'Units', '','Comment', '','StartBit', [ 48;]),struct('Name', 'CS_Temp','Startbit', [ 0;],'SignalSize', [ 8;],'ByteOrder', 'LittleEndian','ValueType', 'UNSIGNED','Class', 'uint8','Signed', [ 0;],'Factor', [ 1;],'Offset', [ 0;],'Min', [ 0;],'Max', [ 255;],'Units', '','Comment', '','StartBit', [ 56;]),struct('Name', 'MotorTempRemaining','Startbit', [ 0;],'SignalSize', [ 16;],'ByteOrder', 'LittleEndian','ValueType', 'SIGNED','Class', 'int16','Signed', [ 1;],'Factor', [ 1;],'Offset', [ 0;],'Min', [ -32768;],'Max', [ 32767;],'Units', 'C','Comment', '','StartBit', [ 16;]),struct('Name', 'InverterTempRemaining','Startbit', [ 0;],'SignalSize', [ 16;],'ByteOrder', 'LittleEndian','ValueType', 'SIGNED','Class', 'int16','Signed', [ 1;],'Factor', [ 1;],'Offset', [ 0;],'Min', [ -32768;],'Max', [ 32767;],'Units', 'C','Comment', '','StartBit', [ 0;])}}
      settings: SourceProductName=Raptor
  Data : Outport  VectorParamsAs1DForOutWhenUnconnected=off
  wires:
  Bus Creator/1 -> Data/1  "MsgName"
  raptor_can_rxmsg/2 -> CANRxField/1  "DC_Link_Voltage"
  raptor_can_rxmsg/3 -> CANRxField1/1  "MotorTempRemaining"
  raptor_can_rxmsg/4 -> CANRxField2/1  "InverterTempRemaining"
  CANRxField2/1 -> Bus Creator/4
  CANRxField1/1 -> Bus Creator/3
  CANRxField/1 -> Bus Creator/2
  CANRxMsgStatus/1 -> Bus Creator/1
  DiagEnbl/1 -> CANRxMsgStatus/1
  raptor_can_rxmsg/1 -> CANRxMsgStatus/2  "Age"

== system VCMGCM1962020b_v2/Fgnd/Sensors/CAN/Other/Power Steering Pump Inverter/PSPInvtrHS4_Fault_Info ==
  DiagEnbl : Inport
  Bus Creator : BusCreator  Inputs=3
  CANRxField : Blocks_lib/CANRxField  typ='uint32'  custom=on  custom_nam=[nam '---']  custom_units='---'
  CANRxField1 : Blocks_lib/CANRxField  typ='uint16'  custom=on  custom_nam=[nam '---']  custom_units='---'
  CANRxMsgStatus : Blocks_lib/CANRxMsgStatus  samptime=samptime  custom=on  custom_nam=[nam '---']  msgnam=PSPInvtrHS4_Fault_Info
  Header : Blocks_lib/Header  width=Landscape  addtext=''
  raptor_can_rxmsg : Raptor_lib/CAN/raptor_can_rxmsg  canDefinition=struct('dbcFile', 'SevconInverter_H_Protocol.dbc','message', 'HS4_Fault_Info','comment', '','signals', {{'CS_Fault','SEQ_Fault','FaultData','FaultCode'}},'enabled', [ 0 0 1 1;],'canBus', 'bus','messageID', [ 421265152;],'idMask', [ 536870656;],'payloadMask', [],'payloadValue', [],'period', [ 0;],'mailbox', 'msgnam','queueSize', [ 1;],'label', [ 1;],'ver', [ 2;],'showID', [ 0;],'showRaw', [ 0;],'fill', [ 0;],'editID', [ 0;],'signalOrder', [ 3;])  canBus=bus  mailbox=msgnam  payloadMask=[]  payloadValue=[]  idMask=hex2dec('1FFFFF00')  queueSize=1  showID=0  label=1  fill=0  id=421265152  showRaw=0  showAge=1  signalOrder=3  signalInfo={{struct('Name', 'CS_Fault','Startbit', [ 0;],'SignalSize', [ 8;],'ByteOrder', 'LittleEndian','ValueType', 'UNSIGNED','Class', 'uint8','Signed', [ 0;],'Factor', [ 1;],'Offset', [ 0;],'Min', [ 0;],'Max', [ 255;],'Units', '','Comment', '','StartBit', [ 56;]),struct('Name', 'SEQ_Fault','Startbit', [ 0;],'SignalSize', [ 8;],'ByteOrder', 'LittleEndian','ValueType', 'UNSIGNED','Class', 'uint8','Signed', [ 0;],'Factor', [ 1;],'Offset', [ 0;],'Min', [ 0;],'Max', [ 255;],'Units', '','Comment', '','StartBit', [ 48;]),struct('Name', 'FaultData','Startbit', [ 0;],'SignalSize', [ 24;],'ByteOrder', 'LittleEndian','ValueType', 'SIGNED','Class', 'int32','Signed', [ 1;],'Factor', [ 1;],'Offset', [ 0;],'Min', [ 0;],'Max', [ 0;],'Units', '','Comment', '','StartBit', [ 16;]),struct('Name', 'FaultCode','Startbit', [ 0;],'SignalSize', [ 16;],'ByteOrder', 'LittleEndian','ValueType', 'SIGNED','Class', 'int16','Signed', [ 1;],'Factor', [ 1;],'Offset', [ 0;],'Min', [ 0;],'Max', [ 0;],'Units', '','Comment', '','StartBit', [ 0;])}}
      settings: SourceProductName=Raptor
  Data : Outport  VectorParamsAs1DForOutWhenUnconnected=off
  wires:
  Bus Creator/1 -> Data/1  "MsgName"
  raptor_can_rxmsg/2 -> CANRxField/1  "FaultData"
  raptor_can_rxmsg/3 -> CANRxField1/1  "FaultCode"
  CANRxField1/1 -> Bus Creator/3
  CANRxField/1 -> Bus Creator/2
  CANRxMsgStatus/1 -> Bus Creator/1
  DiagEnbl/1 -> CANRxMsgStatus/1
  raptor_can_rxmsg/1 -> CANRxMsgStatus/2  "Age"

== system VCMGCM1962020b_v2/Fgnd/Sensors/CAN/Other/Power Steering Pump Inverter/Set Rx IDs ==
  f : TriggerPort  TriggerType=function-call  VariantControl=(inherit)  PortDimensions=1
  Constant : Constant  Value=hex2dec('FF')  OutDataTypeStr=Inherit: Inherit via back propagation
  Data Type Conversion : DataTypeConversion  OutDataTypeStr=uint32
  Header : Blocks_lib/Header  width=Portrait  addtext=''
  raptor_adjustment : Raptor_lib/Data Storage/raptor_adjustment  paramName=[nam 'J1939SA']  nameSource=Parameter  initValue=0  dataType=uint8  storage=Calibration  calDispType=Number  calEnum={'False', 'True'}  calGain=1.0  calOffset=0.0  calMax=inf  calMin=-inf  calFormat=''  calUnit=''  calHelp='J1939 source address'  calAccess=1  calFunction='Sensors | CAN'  calDispHeaders=off  calColHeaders={'Col1' 'Col2' 'Col3'}  calRowHeaders={'Row1' 'Row2' 'Row3'}
      settings: SourceProductName=Raptor
  raptor_can_mailbox_properties : Raptor_lib/CAN/raptor_can_mailbox_properties  mailbox=[nam 'HS1_Torque_Feedback']
      settings: SourceProductName=Raptor
  raptor_can_mailbox_properties1 : Raptor_lib/CAN/raptor_can_mailbox_properties  mailbox=[nam 'HS2_Status_Feedback']
      settings: SourceProductName=Raptor
  raptor_can_mailbox_properties2 : Raptor_lib/CAN/raptor_can_mailbox_properties  mailbox=[nam 'HS3_Temperature_Feedback']
      settings: SourceProductName=Raptor
  raptor_can_mailbox_properties3 : Raptor_lib/CAN/raptor_can_mailbox_properties  mailbox=[nam 'HS4_Fault_Info']
      settings: SourceProductName=Raptor
  wires:
  Constant/1 -> raptor_can_mailbox_properties3/2, raptor_can_mailbox_properties2/2, raptor_can_mailbox_properties1/2, raptor_can_mailbox_properties/2
  Data Type Conversion/1 -> raptor_can_mailbox_properties2/1, raptor_can_mailbox_properties3/1, raptor_can_mailbox_properties1/1, raptor_can_mailbox_properties/1
  raptor_adjustment/1 -> Data Type Conversion/1

== system VCMGCM1962020b_v2/Fgnd/Virtual Sensors/Driver Inputs/Brk/BrkPos/Learn-Up Enable ==
  Data : Inport
  Bus Selector : BusSelector  OutputSignals=VirtualSensors.Spd.VehSpd [kph]
  Header : Blocks_lib/Header  width=Portrait  addtext=''
  Relational Operator : RelationalOperator  Operator=<=  OutDataTypeStr=boolean  RndMeth=Nearest
  raptor_adjustment : Raptor_lib/Data Storage/raptor_adjustment  paramName='BrkPosLearnUpEnblVehSpdThr'  nameSource=Parameter  initValue=0  dataType=double  storage=Calibration  calDispType=Number  calEnum={}  calGain=1.0  calOffset=0.0  calMax=inf  calMin=-inf  calFormat='-1'  calUnit='kph'  calHelp='BrkPosLearn-up strategy enable vehicle speed threshold'  calAccess=1  calFunction='Virtual Sensors | Driver Input'  calDispHeaders=off  calColHeaders={'Col1' 'Col2' 'Col3'}  calRowHeaders={'Row1' 'Row2' 'Row3'}
      settings: SourceProductName=Raptor
  Bool : Outport  VectorParamsAs1DForOutWhenUnconnected=off
  wires:
  Bus Selector/1 -> Relational Operator/1  "<VehSpd [kph]>"
  Data/1 -> Bus Selector/1
  Relational Operator/1 -> Bool/1
  raptor_adjustment/1 -> Relational Operator/2

== system VCMGCM1962020b_v2/Fgnd/Virtual Sensors/PDU/HVBusVolt/HV Bus Voltage/Avg ==
  f : TriggerPort  TriggerType=function-call  VariantControl=Variant  PortDimensions=1
  Data Type Conversion : DataTypeConversion
  Eqn(w/DvdByZeroPro) : Blocks_lib/Eqn(w//DvdByZeroPro)  eqn='u(1) / u(2)'  dmn='u(2)'  dfltval=0
  Header : Blocks_lib/Header  width=Portrait  addtext=''
  Meas&Ovrd : Blocks_lib/Meas&Ovrd  nam=nam  name_source=Parameter  view_as=Number  enum_struct={}  gain=1  min=-inf  max=inf  precision=''  units='V'  help='High-voltage bus voltage'  group=group
  Meas&Ovrd1 : Blocks_lib/Meas&Ovrd  nam=[nam 'Vld']  name_source=Parameter  view_as=Number  enum_struct={}  gain=1  min=-inf  max=inf  precision=''  units='Bool'  help='Data valid'  group='Diagnostics | Data Validity'
  Mux : Mux  Inputs=2
  raptor_data_read : Raptor_lib/Data Storage/raptor_data_read  dataName=[nam 'VldTemp']  dataShape=Scalar  idxSource=Input  idxRow=1  idxCol=1
      settings: SourceProductName=Raptor
  raptor_data_read1 : Raptor_lib/Data Storage/raptor_data_read  dataName=[nam 'Sum']  dataShape=Scalar  idxSource=Input  idxRow=1  idxCol=1
      settings: SourceProductName=Raptor
  raptor_data_read2 : Raptor_lib/Data Storage/raptor_data_read  dataName=[nam 'SumCount']  dataShape=Scalar  idxSource=Input  idxRow=1  idxCol=1
      settings: SourceProductName=Raptor
  Vld : Outport  VectorParamsAs1DForOutWhenUnconnected=off
  V : Outport  Port=2  VectorParamsAs1DForOutWhenUnconnected=off
  wires:
  raptor_data_read1/1 -> Mux/1
  raptor_data_read2/1 -> Data Type Conversion/1
  Mux/1 -> Eqn(w/DvdByZeroPro)/1
  Data Type Conversion/1 -> Mux/2
  Eqn(w/DvdByZeroPro)/1 -> Meas&Ovrd/1
  Meas&Ovrd/1 -> V/1
  Meas&Ovrd1/1 -> Vld/1
  raptor_data_read/1 -> Meas&Ovrd1/1

== system VCMGCM1962020b_v2/Fgnd/Virtual Sensors/PDU/HVBusVolt/HV Bus Voltage/Diag ==
  V : Inport
  f : TriggerPort  TriggerType=function-call  VariantControl=Variant  PortDimensions=1
  Compare To Constant : simulink/Logic and Bit Operations/Compare To Constant  relop=>=  const=2  OutDataTypeStr=boolean
  EvalDiag : Subsystem
  Header : Blocks_lib/Header  width=Portrait  addtext=''
  raptor_data_read : Raptor_lib/Data Storage/raptor_data_read  dataName=[nam 'SumCount']  dataShape=Scalar  idxSource=Input  idxRow=1  idxCol=1
      settings: SourceProductName=Raptor
  wires:
  raptor_data_read/1 -> Compare To Constant/1
  Compare To Constant/1 -> EvalDiag/Enable
  V/1 -> EvalDiag/1(V)

== system VCMGCM1962020b_v2/Fgnd/Virtual Sensors/PDU/HVBusVolt/HV Bus Voltage/Reset ==
  f : TriggerPort  TriggerType=function-call  VariantControl=Variant  PortDimensions=1
  Constant : Constant  Value=uint8(0)
  Constant1 : Constant  Value=double(0)
  Constant2 : Constant  Value=double(0)
  Constant3 : Constant  Value=double(99999)
  Header : Blocks_lib/Header  width=Portrait  addtext=''
  raptor_data_write : Raptor_lib/Data Storage/raptor_data_write  dataName=[nam 'SumCount']  dataShape=Scalar  idxSource=Input Port  idxRow=1  idxCol=1
      settings: SourceProductName=Raptor
  raptor_data_write1 : Raptor_lib/Data Storage/raptor_data_write  dataName=[nam 'Sum']  dataShape=Scalar  idxSource=Input Port  idxRow=1  idxCol=1
      settings: SourceProductName=Raptor
  raptor_data_write2 : Raptor_lib/Data Storage/raptor_data_write  dataName=[nam 'Mx']  dataShape=Scalar  idxSource=Input Port  idxRow=1  idxCol=1
      settings: SourceProductName=Raptor
  raptor_data_write3 : Raptor_lib/Data Storage/raptor_data_write  dataName=[nam 'Mn']  dataShape=Scalar  idxSource=Input Port  idxRow=1  idxCol=1
      settings: SourceProductName=Raptor
  wires:
  Constant/1 -> raptor_data_write/1
  Constant1/1 -> raptor_data_write1/1
  Constant2/1 -> raptor_data_write2/1
  Constant3/1 -> raptor_data_write3/1

== system VCMGCM1962020b_v2/Fgnd/Virtual Sensors/PDU/HVBusVolt/HV Bus Voltage/Sum, Max, Min ==
  note: Note: this temporary data write is here to avoid an update error related to ports.
  Data : Inport
  f : TriggerPort  TriggerType=function-call  VariantControl=Variant  PortDimensions=1
  Data Vectors : Subsystem
  Header : Blocks_lib/Header  width=Portrait  addtext=''
  Logical Operator : Logic  Operator=OR  Inputs=1  AllPortsSameDT=off  OutDataTypeStr=boolean
  Loop : Subsystem  TreatAsAtomicUnit=on
  Width : Width  DataType=uint8
  raptor_data_def : Raptor_lib/Data Storage/raptor_data_def  dataName=[nam 'VldTemp']  initValue=0  dataType=boolean  storage=Volatile (RAM)  calVisible=off  calType=Measurement  calDispType=Number  calEnum={'False', 'True'}  calGain=1.0  calOffset=0  calMin=-inf  calMax=inf  calFormat='-1'  calUnit=''  calHelp=''  calAccess=1  calFunction=raptor_xcp_function(gcb)  calDispHeaders=off  calColHeaders={'Col1' 'Col2' 'Col3'}  calRowHeaders={'Row1' 'Row2' 'Row3'}
      settings: SourceProductName=Raptor
  raptor_data_write : Raptor_lib/Data Storage/raptor_data_write  dataName=[nam 'VldTemp']  dataShape=Scalar  idxSource=Input Port  idxRow=1  idxCol=1
      settings: SourceProductName=Raptor
  wires:
  Width/1 -> Loop/3(N)
  Data Vectors/1(V) -> Loop/1(V)
  Data/1 -> Data Vectors/1(Data)
  Data Vectors/2(Vld) -> Loop/2(Vld), Logical Operator/1, Width/1
  Logical Operator/1 -> raptor_data_write/1

== system VCMGCM1962020b_v2/Fgnd/Virtual Sensors/Vehicle/Range/RangeGain/CntrLoop ==
  Compare To Constant : simulink/Logic and Bit Operations/Compare To Constant  relop=>=  const=rstval  OutDataTypeStr=boolean
  Constant : Constant  Value=init  OutDataTypeStr=uint16
  Header : Blocks_lib/Header  width=Portrait  addtext=''
  Increment Real World : simulink/Additional Math & Discrete/Additional Math: Increment - Decrement/Increment Real World
      settings: SourceProductBaseCode=SL
  Multiport Switch : MultiPortSwitch  DataPortOrder=Zero-based contiguous  Inputs=2  zeroidx=on  InputSameDT=on
  Unit Delay : UnitDelay  InitialCondition=init  SampleTime=-1  HasFrameUpgradeWarning=on
  Count : Outport  VectorParamsAs1DForOutWhenUnconnected=off
  wires:
  Constant/1 -> Multiport Switch/3
  Increment Real World/1 -> Multiport Switch/2
  Compare To Constant/1 -> Multiport Switch/1
  Multiport Switch/1 -> Unit Delay/1, Count/1
  Unit Delay/1 -> Compare To Constant/1, Increment Real World/1

== system VCMGCM1962020b_v2/Fgnd/Virtual Sensors/Vehicle/Range/RangeGain/Moving Average ==
  In1 : Inport
  In2 : Inport  Port=2
  Rst : Inport  Port=3
  Init : Inport  Port=4
  Add : Sum  Inputs=+
  Constant : Constant  Value=5
  Eqn(w/DvdByZeroPro)1 : Blocks_lib/Eqn(w//DvdByZeroPro)  eqn='u(1) / u(2)'  dmn='u(2)'  dfltval=0
  FirstTS : Blocks_lib/FirstTS  SystemSampleTime=-1  VariantActivationTime=update diagram  Latency=0  AutoFrameSizeCalculation=off
  Header : Blocks_lib/Header  width=Portrait  addtext=''
  Multiport Switch : MultiPortSwitch  DataPortOrder=Zero-based contiguous  Inputs=2  zeroidx=on
  Mux : Mux  Inputs=5
  Mux1 : Mux  Inputs=2
  OR : Logic  Operator=OR  AllPortsSameDT=off  OutDataTypeStr=boolean
  OR1 : Logic  Operator=OR  AllPortsSameDT=off  OutDataTypeStr=boolean
  Subsystem : Subsystem
  raptor_data_write : Raptor_lib/Data Storage/raptor_data_write  dataName='RangeGainInit'  dataShape=Scalar  idxSource=Input Port  idxRow=1  idxCol=1
      settings: SourceProductName=Raptor
  raptor_measurement : Raptor_lib/Data Storage/raptor_measurement  paramName='RangeEstGainsTestpoint'  nameSource=Parameter  calDispType=Number  calEnum={'False', 'True'}  calGain=1.0  calOffset=0.0  calMax=inf  calMin=-inf  calFormat='-1'  calUnit=''  calHelp=''  calAccess=1  calFunction=raptor_xcp_function(gcb)  calVisible=on
      settings: SourceProductName=Raptor
  MvAv : Outport
  wires:
  In1/1 -> Multiport Switch/2
  Mux/1 -> raptor_measurement/1, Add/1
  Mux1/1 -> Eqn(w/DvdByZeroPro)1/1
  Add/1 -> Mux1/1
  Constant/1 -> Mux1/2
  Eqn(w/DvdByZeroPro)1/1 -> raptor_data_write/1, MvAv/1
  Init/1 -> Multiport Switch/3, Subsystem/2(Init)
  Multiport Switch/1 -> Subsystem/1(In1), Mux/1
  Subsystem/1(Out1) -> Mux/2
  Subsystem/2(Out2) -> Mux/3
  Subsystem/3(Out3) -> Mux/4
  Subsystem/4(Out4) -> Mux/5
  FirstTS/1 -> OR/1
  Rst/1 -> OR/2
  OR/1 -> OR1/1, Multiport Switch/1
  OR1/1 -> Subsystem/Enable
  In2/1 -> OR1/2
